simulink model "PIDcfAvz"  (R2016a)
settings: Solver=VariableStepAuto  StartTime=0.0  StopTime=20
libraries: fuzblock x1, simulink x1
settings Model: Creator=PC  LastModifiedBy=PC
settings SolverCC: MaxConsecutiveZCs=10000  SolverJacobianMethodControl=FullAnalytical  ZeroCrossControl=DisableAll  ZeroCrossAlgorithm=Adaptive
settings DataIOCC: LimitDataPoints=on  SaveOutput=off  SaveTime=off  Refine=10
settings OptimizationCC: ExpressionDepthLimit=2147483647  LifeSpan=1
settings DebuggingCC: UnderspecifiedInitializationDetection=Classic  MergeDetectMultiDrivingBlocksExec=none  FcnCallInpInsideContextMsg=EnableAllAsWarning  AllowSymbolicDim=off  StateNameClashWarn=warning
settings GRTTargetCC: CombineOutputUpdateFcns=off  GRTInterface=on

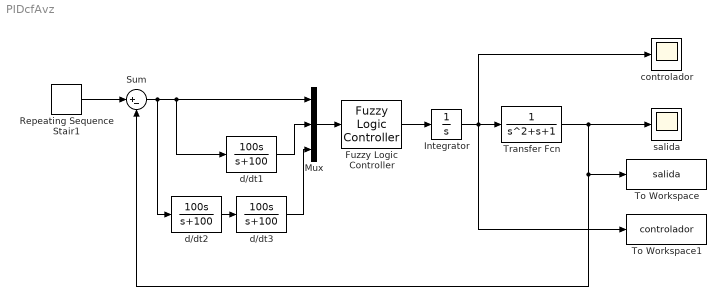
== system PIDcfAvz ==
  Fuzzy Logic Controller : fuzblock/Fuzzy Logic  Controller  fis='PIDdifuso.fis'
  Integrator : Integrator
  Mux : Mux  Inputs=3
  Repeating Sequence Stair1 : simulink/Sources/Repeating Sequence Stair  OutValues=[0 0 1 1 1 1 1 1 0.5 0.5 0.5 0.5 0.5 0.5 0.5 0.5 0.25 0.25 0.25 0.25 0.25 0.25 0.25 1 1].'  tsamp=1  OutMin=[]  OutMax=[]  OutDataTypeStr=double  OutputDataTypeScalingMode=double  OutDataType=fixdt(0,8)  ConRadixGroup=Best Precision: Vector-wise  OutScaling=2^-12
  Sum : Sum  Inputs=|+-
  To Workspace : ToWorkspace  VariableName=salida  SaveFormat=Timeseries  SampleTime=-1
  To Workspace1 : ToWorkspace  VariableName=controlador  SaveFormat=Timeseries  SampleTime=-1
  Transfer Fcn : TransferFcn  Denominator=[1 1 1]
  controlador : Scope
  d/dt1 : TransferFcn  Numerator=[100 0]  Denominator=[1 100]
  d/dt2 : TransferFcn  Numerator=[100 0]  Denominator=[1 100]
  d/dt3 : TransferFcn  Numerator=[100 0]  Denominator=[1 100]
  "salida " : Scope
  wires:
  Repeating Sequence Stair1/1 -> Sum/1
  Transfer Fcn/1 -> "salida "/1, Sum/2, To Workspace/1
  Fuzzy Logic Controller/1 -> Integrator/1
  Mux/1 -> Fuzzy Logic Controller/1
  Sum/1 -> d/dt2/1, Mux/1, d/dt1/1
  d/dt1/1 -> Mux/2
  d/dt2/1 -> d/dt3/1
  d/dt3/1 -> Mux/3
  Integrator/1 -> controlador/1, Transfer Fcn/1, To Workspace1/1
